simulink model "DCMotorControlc2812"  (Simulink 6.5)
settings: Solver=FixedStepDiscrete  StartTime=0.0  StopTime=inf  RelTol=1e-3
PostLoadFcn:
  | runc2812speedcontrolDC
libraries: rtdxBlocks x3, c281xdspchiplib x2, dspbuff3 x2, dspsigops x2, c2000tgtpreflib x1, c28xdmclib x1
settings Model: Creator=maydinli  LastModifiedBy=JacobF  ProdHWDeviceType=TI C2000
settings DataIOCC: SignalLoggingName=logsOut
settings OptimizationCC: InlineInvariantSignals=on  OptimizeModelRefInitCode=on  LifeSpan=1
settings DebuggingCC: CheckExecutionContextPreStartOutputMsg=on  CheckExecutionContextRuntimeOutputMsg=on  MultiTaskDSMMsg=warning  MultiTaskCondExecSysMsg=none  SigSpecEnsureSampleTimeMsg=none  StrictBusMsg=None
settings HardwareCC: ProdBitPerChar=16  ProdBitPerInt=16  ProdIntDivRoundTo=Zero  ProdEndianess=LittleEndian  ProdWordSize=16  ProdHWDeviceType=TI C2000  TargetHWDeviceType=32-bit Generic
settings RTWCC: SystemTargetFile=ti_c2000_ert.tlc  GenCodeOnly=on  TemplateMakefile=ti_c2000_ert.tmf  Description=Embedded Target for TI C2000 DSP (ERT)  ProcessScript=ti_c2000_ert_make_rtw_hook
settings CodeAppCC: IgnoreCustomStorageClasses=off
settings STFCustomTargetCC: TargetFcnLib=ansi_tfl_tmw.mat  GenFloatMathFcnCalls=ANSI_C  ModelReferenceCompliant=off  CombineOutputUpdateFcns=on  ERTCustomFileBanners=on  SupportContinuousTime=off  SupportNonInlinedSFcns=off  SystemTargetFile=ti_c2000_ert.tlc
settings ERTTargetCC: TargetFcnLib=ansi_tfl_tmw.mat  GenFloatMathFcnCalls=ANSI_C  ModelReferenceCompliant=off  InlinedParameterPlacement=NonHierarchical  ERTCustomFileTemplate=example_file_process.tlc

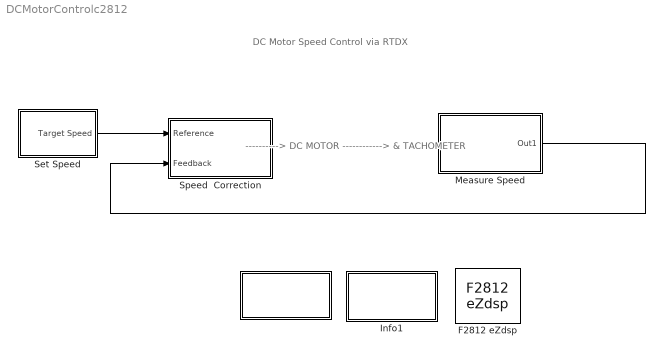
== system DCMotorControlc2812 ==
  note: ----------> DC MOTOR ------------>
      | &
      | TACHOMETER
  note: DC Motor Speed Control via RTDX
  " " : Subsystem
      settings: OpenFcn=runc2812speedcontrolDC
      mask Type: Run demo
      mask Display: disp(sprintf('Build/Reload\n& Run'))
  " Info1" : Subsystem
      settings: OpenFcn=edit runc2812speedcontrolDC;
      mask Display: disp('View Demo\nScript')
  F2812 eZdsp : c2000tgtpreflib/F2812 eZdsp  Tag=C2000 TARGET PREFERENCES BLOCK  SystemSampleTime=-1
  "Measure Speed " : Subsystem  TreatAsAtomicUnit=on  RTWFcnName=Measure_Speed
      settings: RTWSystemCode=Function  RTWFcnNameOpts=User specified
      mask Display: port_label('Output',1,'Speed in RPM');
  Set Speed : Subsystem  TreatAsAtomicUnit=on  RTWFcnName=Set_Speed
      settings: RTWSystemCode=Function  RTWFcnNameOpts=User specified
  Speed  Correction : Subsystem  TreatAsAtomicUnit=on  RTWFcnName=Speed_Correction
      settings: RTWSystemCode=Function  RTWFcnNameOpts=User specified
  wires:
  Set Speed/1(Target Speed) -> Speed  Correction/1(Reference)
  "Measure Speed "/1(Out1) -> Speed  Correction/2(Feedback)

== system DCMotorControlc2812/  ==

== system DCMotorControlc2812/ Info1 ==
  note: This example demonstrates the use of the c2812 ADC block to sample an analog voltage
      | and the c2812 PWM block to generate a pulse waveform. The analog voltage controls the
      | duty cycle of the PWM. Duty cycle change can be observed on the oscilloscope.
      |
      | For results of generated code to match the simulation, apply a pulse waveform toggling
      | between 0.39 and 1.17 V every 2 s.
  note: The code generation portion of this demo requires the following hardware:
      |
      | Spectrum Digital eZdsp F2812
      | Function generator
      | Oscilloscope and probes
      |
      | Connect the function generator output to the ADC input ADCINA0 on the eZdsp F2812.
      | Connect the output of PWM1 on the eZdsp F2812 to the analog input of the oscilloscope.
  note: Setup:
  note: Demo Description:

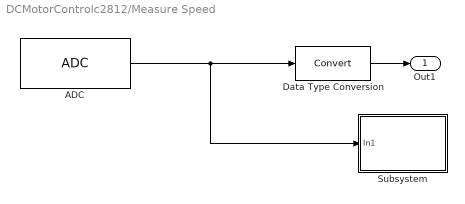
== system DCMotorControlc2812/Measure Speed  ==
  ADC : c281xdspchiplib/ADC  useModule=A  useMode=Sequential  sourceSOC=EVA  Ts=0.01  dType=int32  postInterrupt=off  numConversionsSingle=1  numConversionsDouble=1  conv0=ADCINB0  conv1=ADCINB1  conv2=ADCINB2  conv3=ADCINB3  conv4=ADCINA4  conv5=ADCINA5  conv6=ADCINB6  conv7=ADCINA7  conv8=ADCINB0  conv9=ADCINB1  conv10=ADCINB2  conv11=ADCINB3  conv12=ADCINB4  conv13=ADCINB5  conv14=ADCINB6  conv15=ADCINB7  convAB0=ADCINA0 and ADCINB0  convAB1=ADCINA1 and ADCINB1  convAB2=ADCINA5 and ADCINB5  convAB3=ADCINA1 and ADCINB1  convAB4=ADCINA1 and ADCINB1  convAB5=ADCINA1 and ADCINB1  convAB6=ADCINA1 and ADCINB1  convAB7=ADCINA1 and ADCINB1  convA0=ADCINA0  convA1=ADCINA1  convA2=ADCINA2  convA3=ADCINA3  convA4=ADCINA4  convA5=ADCINA5  convA6=ADCINA6  convA7=ADCINA7  convB0=ADCINB0  convB1=ADCINB1  convB2=ADCINB2  convB3=ADCINB3  convB4=ADCINB4  convB5=ADCINB5  convB6=ADCINB6  convB7=ADCINB7  c28xmultiPort=off
  Data Type Conversion : DataTypeConversion
  Subsystem : Subsystem
      mask Display: disp('Take Samples');
  Out1 : Outport
  wires:
  Data Type Conversion/1 -> Out1/1
  ADC/1 -> Data Type Conversion/1, Subsystem/1(In1)

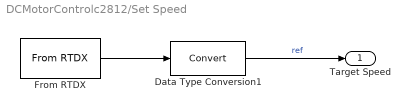
== system DCMotorControlc2812/Set Speed ==
  Data Type Conversion1 : DataTypeConversion  OutDataTypeMode=Specify via dialog  OutDataType=sfix(32)  OutScaling=2^-15
  From RTDX : rtdxBlocks/From RTDX  channelNameStr=ichan1  isBlocking=off  icMaskVar=1000  Ts=0.01  dims=[1 1]  isFrame=off  dType=int32  isChannelEnabled=on  isHighSpeedRTDXUsed=off
  Target Speed : Outport
  wires:
  Data Type Conversion1/1 -> Target Speed/1  "ref"
  From RTDX/1 -> Data Type Conversion1/1

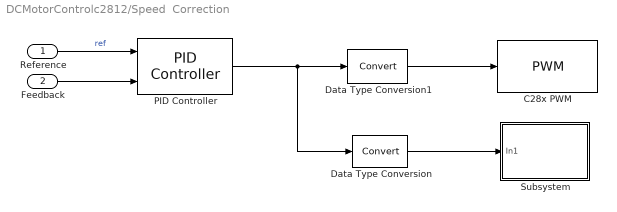
== system DCMotorControlc2812/Speed  Correction ==
  Reference : Inport
  Feedback : Inport  Port=2
  C28x PWM : c281xdspchiplib/PWM  useModule=A  timerSource=Specify via dialog  timerPeriod=4096  waveformType=Symmetric  periodUnits=Clock cycles  unit1Status=on  unit1Source=Input port  unit1Value=18500  unit2Status=off  unit2Source=Specify via dialog  unit2Value=18500  unit3Status=off  unit3Source=Specify via dialog  unit3Value=18500  dutyCycleUnits=Clock cycles  logicSource=Specify via dialog  unit1_1Logic=Active low  unit1_2Logic=Active low  unit2_1Logic=Active high  unit2_2Logic=Active low  unit3_1Logic=Active high  unit3_2Logic=Active low  enableDeadband1=off  enableDeadband2=off  enableDeadband3=off  deadbandPrescaler=16  deadbandPeriodSource=Specify via dialog  deadbandPeriod=12  adcstartEvent=Period interrupt
  Data Type Conversion : DataTypeConversion  OutDataTypeMode=int32  RndMeth=Nearest  SaturateOnIntegerOverflow=on
  Data Type Conversion1 : DataTypeConversion  OutDataTypeMode=uint16  RndMeth=Nearest  SaturateOnIntegerOverflow=on
  PID Controller : c28xdmclib/PID Controller  proportionalGain=0.1  integralGain=0.9  correctionGain=0.3  derivativeGain=1.2  minOutput=1000  maxOutput=4000
  Subsystem : Subsystem
      mask Display: disp('Take Samples');
  wires:
  PID Controller/1 -> Data Type Conversion1/1, Data Type Conversion/1
  Data Type Conversion/1 -> Subsystem/1(In1)
  Reference/1 -> PID Controller/1  "ref"
  Feedback/1 -> PID Controller/2
  Data Type Conversion1/1 -> C28x PWM/1

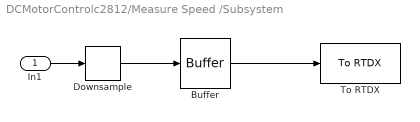
== system DCMotorControlc2812/Measure Speed /Subsystem ==
  In1 : Inport
  Buffer : dspbuff3/Buffer  N=50  V=49  ic=0
  Downsample : dspsigops/Downsample  N=10  phase=0  ic=0  smode=Allow multirate  fmode=Maintain input frame size
  To RTDX : rtdxBlocks/To RTDX  channelNameStr=ochan1  isBlocking=on  isChannelEnabled=on
  wires:
  Buffer/1 -> To RTDX/1
  Downsample/1 -> Buffer/1
  In1/1 -> Downsample/1

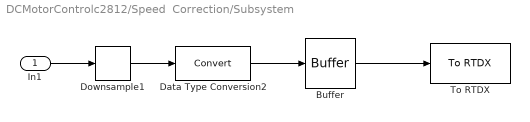
== system DCMotorControlc2812/Speed  Correction/Subsystem ==
  In1 : Inport
  Buffer : dspbuff3/Buffer  N=50  V=49  ic=0
  Data Type Conversion2 : DataTypeConversion  OutDataTypeMode=int32
  Downsample1 : dspsigops/Downsample  N=10  phase=0  ic=0  smode=Allow multirate  fmode=Maintain input frame size
  To RTDX : rtdxBlocks/To RTDX  channelNameStr=ochan2  isBlocking=on  isChannelEnabled=on
  wires:
  In1/1 -> Downsample1/1
  Downsample1/1 -> Data Type Conversion2/1
  Buffer/1 -> To RTDX/1
  Data Type Conversion2/1 -> Buffer/1
